simulink model "networkanalyzer"  (R2012b)
settings: Solver=ode3  SolverMode=SingleTasking  StartTime=0.0  StopTime=50000  RelTol=1e-3
libraries: xbsIndex_r4 x1097, casper_library_flow_control x33, casper_library_misc x21, xps_library x10
(part 2 of 8)

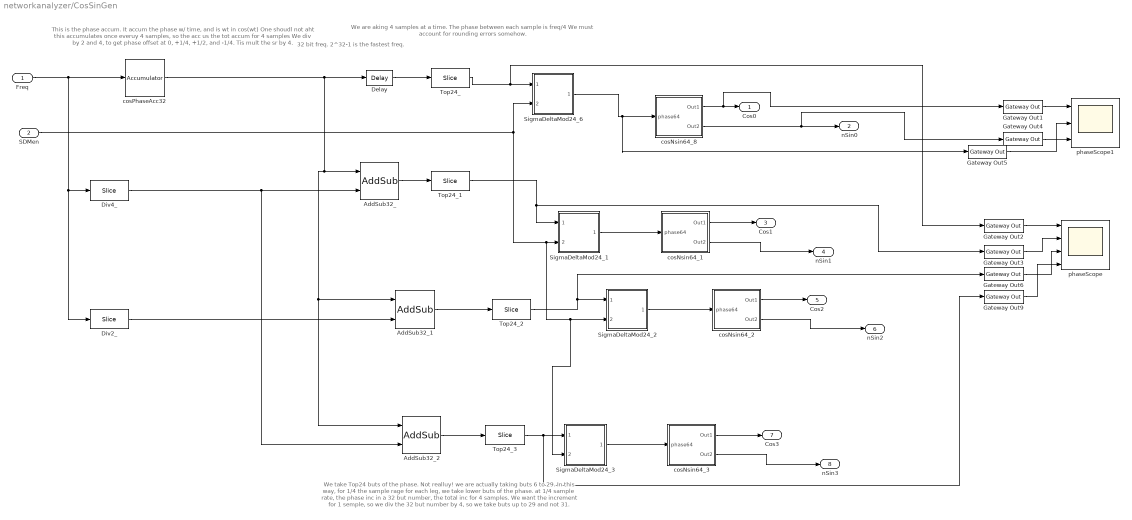
== system networkanalyzer/CosSinGen ==
  note: We take Top24 buts of the phase.
      | Not realluy! we are actually taking buts 6 to 29. In this way,
      | for 1/4 the sample rage for each leg, we take lower buts
      | of the phase. at 1/4 sample rate, the phase inc in a 32 but number,
      | the total inc for 4 samples. We want the increment for 1 semple, so
      | we div the 32 but number by 4, so we take buts up to 29 and not 31.
  note: This is the phase accum. It accum the phase w/ time, and is wt in cos(wt)
      | One shoudl not aht this accumulates once everuy 4 samples, so the acc us the tot accum for 4 samples
      | We div by 2 and 4, to get phase offset at 0, +1/4, +1/2, and -1/4. Tis mult the sr by 4.
  note: 32 bit freq. 2^32-1 is the fastest freq.
  note: We are aking 4 samples at a time.
      | The phase between each sample is freq/4
      | We must account for rounding errors somehow.
  Freq : Inport
  SDMen : Inport  Port=2
  AddSub32_ : xbsIndex_r4/AddSub  mode=Addition  use_carryin=off  use_carryout=off  en=off  latency=2  precision=User Defined  arith_type=Unsigned  n_bits=32  bin_pt=0  quantization=Truncate  overflow=Wrap  dbl_ovrd=off  use_behavioral_HDL=off  hw_selection=Fabric  pipelined=off  block_type=addsub
  AddSub32_1 : xbsIndex_r4/AddSub  mode=Addition  use_carryin=off  use_carryout=off  en=off  latency=2  precision=User Defined  arith_type=Unsigned  n_bits=32  bin_pt=0  quantization=Truncate  overflow=Wrap  dbl_ovrd=off  use_behavioral_HDL=off  hw_selection=Fabric  pipelined=off  block_type=addsub
  AddSub32_2 : xbsIndex_r4/AddSub  mode=Subtraction  use_carryin=off  use_carryout=off  en=off  latency=2  precision=User Defined  arith_type=Unsigned  n_bits=32  bin_pt=0  quantization=Truncate  overflow=Wrap  dbl_ovrd=off  use_behavioral_HDL=off  hw_selection=Fabric  pipelined=off  block_type=addsub
  Delay : xbsIndex_r4/Delay  rst=off  infoeditControl=Selection of Reset will increase slice count due to use of real FFs and instead of SRLs  en=off  latency=2  dbl_ovrd=off  reg_retiming=off  block_type=delay
  Div2_ : xbsIndex_r4/Slice  nbits=31  boolean_output=off  mode=Two Bit Locations  bit1=0  base1=MSB of Input  bit0=1  base0=LSB of Input  dbl_ovrd=off  block_type=slice
  Div4_ : xbsIndex_r4/Slice  nbits=30  boolean_output=off  mode=Two Bit Locations  bit1=0  base1=MSB of Input  bit0=2  base0=LSB of Input  dbl_ovrd=off  block_type=slice
  Gateway Out{1..6,9} (7 alike) : xbsIndex_r4/Gateway Out  inherit_from_input=off  hdl_port=off  timing_constraint=None  locs_specified=off  LOCs={}  UseAsDAC=off  DACChannel='1'  block_type=gatewayout
  SigmaDeltaMod24_1 : Subsystem
  SigmaDeltaMod24_2 : Subsystem
  SigmaDeltaMod24_3 : Subsystem
  SigmaDeltaMod24_6 : Subsystem
  Top24_{,1..3} (4 alike) : xbsIndex_r4/Slice  nbits=24  boolean_output=off  mode=Two Bit Locations  bit1=0  base1=MSB of Input  bit0=6  base0=LSB of Input  dbl_ovrd=off  block_type=slice
  cosNsin64_1 : Subsystem
  cosNsin64_2 : Subsystem
  cosNsin64_3 : Subsystem
  cosNsin64_8 : Subsystem
  cosPhaseAcc32 : xbsIndex_r4/Accumulator  operation=Add  n_bits=32  overflow=Wrap  scale=1  rst=off  hasbypass=off  en=off  dbl_ovrd=off  use_behavioral_HDL=on  implementation=Fabric  block_type=accum
  phaseScope : Scope  NumInputPorts=4
      settings: TimeRange=5000  YMin=0~-5~-5~-5  YMax=300000~5~5~5  SaveName=ScopeData3  MaxDataPoints=10000
  phaseScope1 : Scope  NumInputPorts=3
      settings: TimeRange=5000  YMin=0~-5~-5  YMax=300000~5~5  SaveName=ScopeData6  MaxDataPoints=10000
  Cos0 : Outport
  nSin0 : Outport  Port=2
  Cos1 : Outport  Port=3
  nSin1 : Outport  Port=4
  Cos2 : Outport  Port=5
  nSin2 : Outport  Port=6
  Cos3 : Outport  Port=7
  nSin3 : Outport  Port=8
  wires:
  cosNsin64_1/1(Out1) -> Cos1/1
  cosNsin64_8/2(Out2) -> Gateway Out4/1, nSin0/1
  SigmaDeltaMod24_6/1(DataOut) -> Gateway Out5/1, cosNsin64_8/1(phase64)
  cosNsin64_1/2(Out2) -> nSin1/1
  SDMen/1 -> SigmaDeltaMod24_1/2(SDMEn), SigmaDeltaMod24_3/2(SDMEn), SigmaDeltaMod24_2/2(SDMEn), SigmaDeltaMod24_6/2(SDMEn)
  SigmaDeltaMod24_1/1(DataOut) -> cosNsin64_1/1(phase64)
  Freq/1 -> cosPhaseAcc32/1, Div2_/1, Div4_/1
  Top24_/1 -> Gateway Out2/1, SigmaDeltaMod24_6/1(DataIn)
  cosNsin64_2/1(Out1) -> Cos2/1
  cosNsin64_2/2(Out2) -> nSin2/1
  Top24_2/1 -> SigmaDeltaMod24_2/1(DataIn), Gateway Out6/1
  cosNsin64_3/1(Out1) -> Cos3/1
  cosNsin64_3/2(Out2) -> nSin3/1
  SigmaDeltaMod24_3/1(DataOut) -> cosNsin64_3/1(phase64)
  cosPhaseAcc32/1 -> Delay/1, AddSub32_1/1, AddSub32_2/1, AddSub32_/1
  Div4_/1 -> AddSub32_2/2, AddSub32_/2
  AddSub32_/1 -> Top24_1/1
  Top24_1/1 -> SigmaDeltaMod24_1/1(DataIn), Gateway Out3/1
  AddSub32_1/1 -> Top24_2/1
  Div2_/1 -> AddSub32_1/2
  Delay/1 -> Top24_/1
  AddSub32_2/1 -> Top24_3/1
  Gateway Out2/1 -> phaseScope/1
  Gateway Out3/1 -> phaseScope/2
  Gateway Out6/1 -> phaseScope/3
  Gateway Out9/1 -> phaseScope/4
  SigmaDeltaMod24_2/1(DataOut) -> cosNsin64_2/1(phase64)
  Top24_3/1 -> SigmaDeltaMod24_3/1(DataIn), Gateway Out9/1
  cosNsin64_8/1(Out1) -> Gateway Out1/1, Cos0/1
  Gateway Out1/1 -> phaseScope1/1
  Gateway Out4/1 -> phaseScope1/3
  Gateway Out5/1 -> phaseScope1/2

== system networkanalyzer/DFTMem1 ==
  Start : Inport
  Sel : Inport  Port=2
  Src0 : Inport  Port=3
  Src1 : Inport  Port=4
  Src2 : Inport  Port=5
  Src3 : Inport  Port=6
  WE : Inport  Port=7
  WE1 : Inport  Port=8
  Src4 : Inport  Port=9
  Src5 : Inport  Port=10
  Src6 : Inport  Port=11
  Src7 : Inport  Port=12
  Logical : xbsIndex_r4/Logical  logical_function=OR  inputs=2  en=off  latency=0  precision=Full  arith_type=Unsigned  n_bits=16  bin_pt=0  align_bp=on  dbl_ovrd=off  block_type=logical
  MemRecord : Subsystem
  Mux : xbsIndex_r4/Mux  inputs=8  en=off  latency=0  precision=Full  arith_type=Unsigned  n_bits=16  bin_pt=14  quantization=Truncate  overflow=Wrap  dbl_ovrd=off  block_type=mux
  edge_detect : casper_library_misc/edge_detect  edge=Rising  polarity=Active High  x_in=[0 0.08 0.08 0.16 0.16 0.24 0.24 0.32 0.32 0.4]  y_in="[-1 -1  1  1  1  1  1  1  1  1]"  x_out=[0.6 0.68 0.68 0.76 0.76 0.84 0.84 0.92 0.92 1]  y_out="[-1 -1  1  1 -1 -1 -1 -1 -1 -1]"
  Out1 : Outport
  wires:
  Src2/1 -> Mux/4
  Sel/1 -> Mux/1
  edge_detect/1 -> Logical/2
  WE/1 -> Logical/1
  Src0/1 -> Mux/2
  Src1/1 -> Mux/3
  Src3/1 -> Mux/5
  WE1/1 -> edge_detect/1
  MemRecord/1(memDone) -> Out1/1
  Mux/1 -> MemRecord/2(DataIn)
  Start/1 -> MemRecord/1(Start)
  Logical/1 -> MemRecord/3(WE)
  Src4/1 -> Mux/6
  Src5/1 -> Mux/7
  Src6/1 -> Mux/8
  Src7/1 -> Mux/9

== system networkanalyzer/DFTMem2 ==
  Start : Inport
  Sel : Inport  Port=2
  Src0 : Inport  Port=3
  Src1 : Inport  Port=4
  Src2 : Inport  Port=5
  Src3 : Inport  Port=6
  WE : Inport  Port=7
  WE1 : Inport  Port=8
  Src4 : Inport  Port=9
  Src5 : Inport  Port=10
  Src6 : Inport  Port=11
  Src7 : Inport  Port=12
  Logical : xbsIndex_r4/Logical  logical_function=OR  inputs=2  en=off  latency=0  precision=Full  arith_type=Unsigned  n_bits=16  bin_pt=0  align_bp=on  dbl_ovrd=off  block_type=logical
  MemRecord : Subsystem
  Mux : xbsIndex_r4/Mux  inputs=8  en=off  latency=0  precision=Full  arith_type=Unsigned  n_bits=16  bin_pt=14  quantization=Truncate  overflow=Wrap  dbl_ovrd=off  block_type=mux
  edge_detect : casper_library_misc/edge_detect  edge=Rising  polarity=Active High  x_in=[0 0.08 0.08 0.16 0.16 0.24 0.24 0.32 0.32 0.4]  y_in="[-1 -1  1  1  1  1  1  1  1  1]"  x_out=[0.6 0.68 0.68 0.76 0.76 0.84 0.84 0.92 0.92 1]  y_out="[-1 -1  1  1 -1 -1 -1 -1 -1 -1]"
  Out1 : Outport
  wires:
  Src2/1 -> Mux/4
  Sel/1 -> Mux/1
  edge_detect/1 -> Logical/2
  WE/1 -> Logical/1
  Src0/1 -> Mux/2
  Src1/1 -> Mux/3
  Src3/1 -> Mux/5
  WE1/1 -> edge_detect/1
  MemRecord/1(memDone) -> Out1/1
  Mux/1 -> MemRecord/2(DataIn)
  Start/1 -> MemRecord/1(Start)
  Logical/1 -> MemRecord/3(WE)
  Src4/1 -> Mux/6
  Src5/1 -> Mux/7
  Src6/1 -> Mux/8
  Src7/1 -> Mux/9

== system networkanalyzer/DFTMem3 ==
  Start : Inport
  Sel : Inport  Port=2
  Src0 : Inport  Port=3
  Src1 : Inport  Port=4
  Src2 : Inport  Port=5
  Src3 : Inport  Port=6
  WE : Inport  Port=7
  WE1 : Inport  Port=8
  Src4 : Inport  Port=9
  Src5 : Inport  Port=10
  Src6 : Inport  Port=11
  Src7 : Inport  Port=12
  Logical : xbsIndex_r4/Logical  logical_function=OR  inputs=2  en=off  latency=0  precision=Full  arith_type=Unsigned  n_bits=16  bin_pt=0  align_bp=on  dbl_ovrd=off  block_type=logical
  MemRecord : Subsystem
  Mux : xbsIndex_r4/Mux  inputs=8  en=off  latency=0  precision=Full  arith_type=Unsigned  n_bits=16  bin_pt=14  quantization=Truncate  overflow=Wrap  dbl_ovrd=off  block_type=mux
  edge_detect : casper_library_misc/edge_detect  edge=Rising  polarity=Active High  x_in=[0 0.08 0.08 0.16 0.16 0.24 0.24 0.32 0.32 0.4]  y_in="[-1 -1  1  1  1  1  1  1  1  1]"  x_out=[0.6 0.68 0.68 0.76 0.76 0.84 0.84 0.92 0.92 1]  y_out="[-1 -1  1  1 -1 -1 -1 -1 -1 -1]"
  Out1 : Outport
  wires:
  Src2/1 -> Mux/4
  Sel/1 -> Mux/1
  edge_detect/1 -> Logical/2
  WE/1 -> Logical/1
  Src0/1 -> Mux/2
  Src1/1 -> Mux/3
  Src3/1 -> Mux/5
  WE1/1 -> edge_detect/1
  MemRecord/1(memDone) -> Out1/1
  Mux/1 -> MemRecord/2(DataIn)
  Start/1 -> MemRecord/1(Start)
  Logical/1 -> MemRecord/3(WE)
  Src4/1 -> Mux/6
  Src5/1 -> Mux/7
  Src6/1 -> Mux/8
  Src7/1 -> Mux/9

== system networkanalyzer/DFTMem4 ==
  Start : Inport
  Sel : Inport  Port=2
  Src0 : Inport  Port=3
  Src1 : Inport  Port=4
  Src2 : Inport  Port=5
  Src3 : Inport  Port=6
  WE : Inport  Port=7
  WE1 : Inport  Port=8
  Src4 : Inport  Port=9
  Src5 : Inport  Port=10
  Src6 : Inport  Port=11
  Src7 : Inport  Port=12
  Logical : xbsIndex_r4/Logical  logical_function=OR  inputs=2  en=off  latency=0  precision=Full  arith_type=Unsigned  n_bits=16  bin_pt=0  align_bp=on  dbl_ovrd=off  block_type=logical
  MemRecord : Subsystem
  Mux : xbsIndex_r4/Mux  inputs=8  en=off  latency=0  precision=Full  arith_type=Unsigned  n_bits=16  bin_pt=14  quantization=Truncate  overflow=Wrap  dbl_ovrd=off  block_type=mux
  edge_detect : casper_library_misc/edge_detect  edge=Rising  polarity=Active High  x_in=[0 0.08 0.08 0.16 0.16 0.24 0.24 0.32 0.32 0.4]  y_in="[-1 -1  1  1  1  1  1  1  1  1]"  x_out=[0.6 0.68 0.68 0.76 0.76 0.84 0.84 0.92 0.92 1]  y_out="[-1 -1  1  1 -1 -1 -1 -1 -1 -1]"
  Out1 : Outport
  wires:
  Src2/1 -> Mux/4
  Sel/1 -> Mux/1
  edge_detect/1 -> Logical/2
  WE/1 -> Logical/1
  Src0/1 -> Mux/2
  Src1/1 -> Mux/3
  Src3/1 -> Mux/5
  WE1/1 -> edge_detect/1
  MemRecord/1(memDone) -> Out1/1
  Mux/1 -> MemRecord/2(DataIn)
  Start/1 -> MemRecord/1(Start)
  Logical/1 -> MemRecord/3(WE)
  Src4/1 -> Mux/6
  Src5/1 -> Mux/7
  Src6/1 -> Mux/8
  Src7/1 -> Mux/9

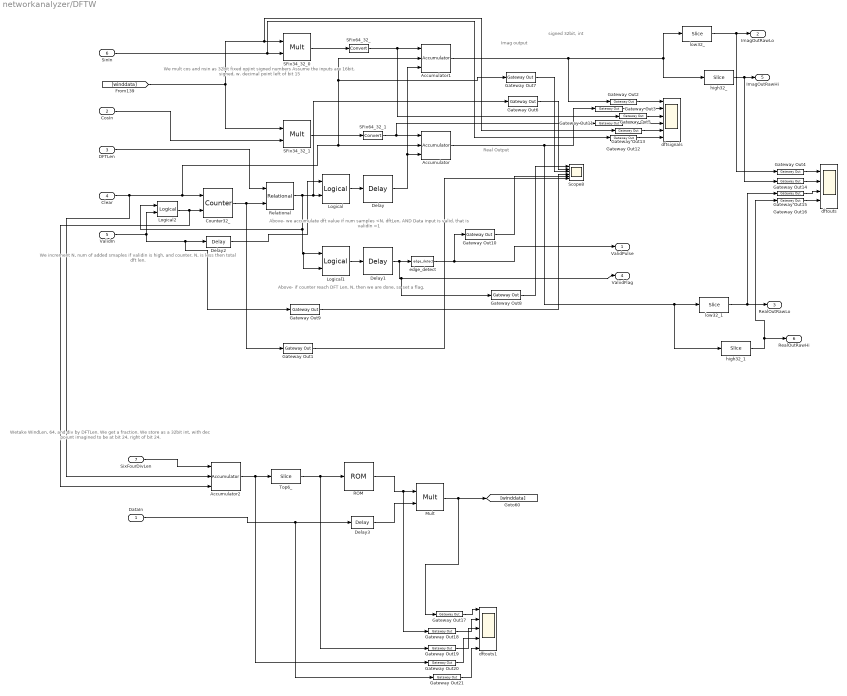
== system networkanalyzer/DFTW ==
  note: Wetake WindLen, 64, and div by DFTLen.
      | We get a fraction. We store as a 32bit int, with dec poiunt imagined to
      | be at bit 24, right of bit 24.
  note: Real Output
  note: Imag output
  note: We mult cos and nsin as 32bit fixed opjint signed numbers
      | Assume the inputs are 16bit, signed, w. decimal point left of bit 15
  note: Above- if counter reach DFT Len, N, then we are done, so set a flag.
  note: Above- we accumulate dft value if num samples <N, dftLen, AND
      | Data input is valid, that is validIn =1
  note: We increment N, num of added smaples if validin is high, and
      | counter, N, is less then total dft len.
  note: signed 32bit, int
  DataIn : Inport
  CosIn : Inport  Port=2
  DFTLen : Inport  Port=3
  Clear : Inport  Port=4
  ValidIn : Inport  Port=5
  SinIn : Inport  Port=6
  SixFourDivLen : Inport  Port=7
  Accumulator : xbsIndex_r4/Accumulator  operation=Add  n_bits=64  overflow=Wrap  scale=1  rst=on  hasbypass=off  en=on  dbl_ovrd=off  use_behavioral_HDL=on  implementation=Fabric  block_type=accum
  Accumulator1 : xbsIndex_r4/Accumulator  operation=Add  n_bits=64  overflow=Wrap  scale=1  rst=on  hasbypass=off  en=on  dbl_ovrd=off  use_behavioral_HDL=on  implementation=Fabric  block_type=accum
  Accumulator2 : xbsIndex_r4/Accumulator  operation=Add  n_bits=32  overflow=Wrap  scale=1  rst=on  hasbypass=off  en=on  dbl_ovrd=off  use_behavioral_HDL=on  implementation=Fabric  block_type=accum
  Counter32_ : xbsIndex_r4/Counter  cnt_type=Free Running  cnt_to=Inf  operation=Up  start_count=0  cnt_by_val=1  arith_type=Unsigned  n_bits=32  bin_pt=0  load_pin=off  rst=on  en=on  explicit_period=on  period=1  dbl_ovrd=off  use_behavioral_HDL=off  implementation=Fabric  block_type=counter
  Delay : xbsIndex_r4/Delay  rst=off  infoeditControl=Selection of Reset will increase slice count due to use of real FFs and instead of SRLs  en=off  latency=2  dbl_ovrd=off  reg_retiming=off  block_type=delay
  Delay1 : xbsIndex_r4/Delay  rst=off  infoeditControl=Selection of Reset will increase slice count due to use of real FFs and instead of SRLs  en=off  latency=2  dbl_ovrd=off  reg_retiming=off  block_type=delay
  Delay2 : xbsIndex_r4/Delay  rst=off  infoeditControl=Selection of Reset will increase slice count due to use of real FFs and instead of SRLs  en=off  latency=2  dbl_ovrd=off  reg_retiming=off  block_type=delay
  Delay3 : xbsIndex_r4/Delay  rst=off  infoeditControl=Selection of Reset will increase slice count due to use of real FFs and instead of SRLs  en=off  latency=1  dbl_ovrd=off  reg_retiming=off  block_type=delay
  Gateway Out{1..21} (21 alike) : xbsIndex_r4/Gateway Out  inherit_from_input=off  hdl_port=off  timing_constraint=None  locs_specified=off  LOCs={}  UseAsDAC=off  DACChannel='1'  block_type=gatewayout
  Logical : xbsIndex_r4/Logical  logical_function=AND  inputs=2  en=off  latency=1  precision=Full  arith_type=Unsigned  n_bits=16  bin_pt=0  align_bp=on  dbl_ovrd=off  block_type=logical
  Logical1 : xbsIndex_r4/Logical  logical_function=NAND  inputs=2  en=off  latency=1  precision=Full  arith_type=Unsigned  n_bits=16  bin_pt=0  align_bp=on  dbl_ovrd=off  block_type=logical
  Logical2 : xbsIndex_r4/Logical  logical_function=AND  inputs=2  en=off  latency=0  precision=Full  arith_type=Unsigned  n_bits=16  bin_pt=0  align_bp=on  dbl_ovrd=off  block_type=logical
  Mult : xbsIndex_r4/Mult  precision=User Defined  arith_type="Signed  (2's comp)"  n_bits=16  bin_pt=15  quantization=Truncate  overflow=Wrap  en=off  latency=3  dbl_ovrd=off  use_behavioral_HDL=off  opt=Speed  use_embedded=on  optimum_pipeline=off  pipeline=on  use_rpm=on  placement_style=Triangular  block_type=mult
  ROM : xbsIndex_r4/ROM  depth=64  initVector=0.5-0.5*cos(2*pi*(0:63)/63)  distributed_mem=Block RAM  rst=off  init_reg=0  en=off  latency=1  gui_display_data_type=Fixed-point  arith_type="Signed  (2's comp)"  n_bits=16  bin_pt=15  preci_type=Single  exp_width=8  frac_width=24  dbl_ovrd=off  optimize=Area  use_rpm=on  block_type=sprom
  Relational : xbsIndex_r4/Relational  mode=a>=b  en=off  latency=1  dbl_ovrd=off  block_type=relational
  SFix34_32_0 : xbsIndex_r4/Mult  precision=User Defined  arith_type="Signed  (2's comp)"  n_bits=34  bin_pt=32  quantization=Truncate  overflow=Saturate  en=off  latency=4  dbl_ovrd=off  use_behavioral_HDL=off  opt=Speed  use_embedded=on  optimum_pipeline=off  pipeline=on  use_rpm=on  placement_style=Triangular  block_type=mult
  SFix34_32_1 : xbsIndex_r4/Mult  precision=User Defined  arith_type="Signed  (2's comp)"  n_bits=34  bin_pt=32  quantization=Truncate  overflow=Saturate  en=off  latency=4  dbl_ovrd=off  use_behavioral_HDL=off  opt=Speed  use_embedded=on  optimum_pipeline=off  pipeline=on  use_rpm=on  placement_style=Triangular  block_type=mult
  SFix64_32_ : xbsIndex_r4/Convert  gui_display_data_type=Fixed-point  arith_type="Signed  (2's comp)"  n_bits=64  bin_pt=32  float_type=Single  exp_bits=8  fraction_bits=24  quantization=Truncate  overflow=Wrap  en=off  latency=0  dbl_ovrd=off  pipeline=off  block_type=convert
  SFix64_32_1 : xbsIndex_r4/Convert  gui_display_data_type=Fixed-point  arith_type="Signed  (2's comp)"  n_bits=64  bin_pt=32  float_type=Single  exp_bits=8  fraction_bits=24  quantization=Truncate  overflow=Wrap  en=off  latency=0  dbl_ovrd=off  pipeline=off  block_type=convert
  Scope8 : Scope  NumInputPorts=6
      settings: YMin=0~-5~-5~-5~-5~-5  YMax=300000~5~5~5~5~5  SaveName=ScopeData18  MaxDataPoints=10000
  Top6_ : xbsIndex_r4/Slice  nbits=6  boolean_output=off  mode=Upper Bit Location + Width  bit1=0  base1=MSB of Input  bit0=0  base0=LSB of Input  dbl_ovrd=off  block_type=slice
  dftouts : Scope  NumInputPorts=4
      settings: YMin=0~-5~-5~-5  YMax=300000~5~5~5  SaveName=ScopeData5  MaxDataPoints=10000
  dftouts1 : Scope  NumInputPorts=5
      settings: YMin=-1~0~0~0~-1  YMax=5.55112e-17~1~70~5e+09~0  MaxDataPoints=10000
  dftsignals : Scope  NumInputPorts=6
      settings: YMin=0~-5~-5~-5~-5~-5  YMax=300000~5~5~5~5~5  SaveName=ScopeData4  MaxDataPoints=10000
  edge_detect : casper_library_misc/edge_detect  edge=Rising  polarity=Active High  x_in=[0 0.08 0.08 0.16 0.16 0.24 0.24 0.32 0.32 0.4]  y_in="[-1 -1  1  1  1  1  1  1  1  1]"  x_out=[0.6 0.68 0.68 0.76 0.76 0.84 0.84 0.92 0.92 1]  y_out="[-1 -1  1  1 -1 -1 -1 -1 -1 -1]"
  high32_ : xbsIndex_r4/Slice  nbits=32  boolean_output=off  mode=Lower Bit Location + Width  bit1=-32  base1=MSB of Input  bit0=32  base0=LSB of Input  dbl_ovrd=off  block_type=slice
  high32_1 : xbsIndex_r4/Slice  nbits=32  boolean_output=off  mode=Lower Bit Location + Width  bit1=-31  base1=MSB of Input  bit0=32  base0=LSB of Input  dbl_ovrd=off  block_type=slice
  low32_ : xbsIndex_r4/Slice  nbits=32  boolean_output=off  mode=Lower Bit Location + Width  bit1=-31  base1=MSB of Input  bit0=0  base0=LSB of Input  dbl_ovrd=off  block_type=slice
  low32_1 : xbsIndex_r4/Slice  nbits=32  boolean_output=off  mode=Lower Bit Location + Width  bit1=-31  base1=MSB of Input  bit0=0  base0=LSB of Input  dbl_ovrd=off  block_type=slice
  ValidPulse : Outport
  ImagOutRawLo : Outport  Port=2
  RealOutRawLo : Outport  Port=3
  ValiidFlag : Outport  Port=4
  ImagOutRawHi : Outport  Port=5
  RealOutRawHi : Outport  Port=6
  wires:
  SFix34_32_1/1 -> SFix64_32_1/1
  Relational/1 -> Logical2/1, Logical1/2, Logical1/1, Gateway Out6/1, Logical/2
  Counter32_/1 -> Gateway Out1/1, Relational/2
  [winddata] -> SFix34_32_1/1, Gateway Out13/1, SFix34_32_0/1
  CosIn/1 -> SFix34_32_1/2
  DFTLen/1 -> Relational/1
  ValidIn/1 -> Logical2/2, Gateway Out9/1, Delay2/1
  Clear/1 -> Accumulator2/2, Gateway Out7/1, Accumulator1/2, Accumulator/2, Counter32_/1
  SinIn/1 -> Gateway Out12/1, SFix34_32_0/2
  Logical/1 -> Delay/1
  Delay/1 -> Accumulator1/3, Accumulator/3
  Logical1/1 -> Delay1/1
  Delay1/1 -> Gateway Out8/1, ValiidFlag/1, edge_detect/1
  edge_detect/1 -> Gateway Out10/1, ValidPulse/1
  Gateway Out6/1 -> Scope8/2
  Gateway Out7/1 -> Scope8/3
  Gateway Out8/1 -> Scope8/1
  Gateway Out9/1 -> Scope8/4
  Gateway Out10/1 -> Scope8/5
  Gateway Out1/1 -> Scope8/6
  Logical2/1 -> Accumulator2/3, Counter32_/2
  Delay2/1 -> Logical/1
  SFix34_32_0/1 -> SFix64_32_/1
  Gateway Out2/1 -> dftsignals/1
  Gateway Out3/1 -> dftsignals/2
  Gateway Out5/1 -> dftsignals/3
  Gateway Out13/1 -> dftsignals/5
  Gateway Out11/1 -> dftsignals/4
  Gateway Out12/1 -> dftsignals/6
  SFix64_32_/1 -> Gateway Out5/1, Accumulator1/1
  SFix64_32_1/1 -> Gateway Out11/1, Accumulator/1
  Accumulator1/1 -> Gateway Out2/1, high32_/1, low32_/1
  Accumulator/1 -> high32_1/1, low32_1/1, Gateway Out3/1
  low32_/1 -> Gateway Out4/1, ImagOutRawLo/1
  high32_/1 -> Gateway Out14/1, ImagOutRawHi/1
  low32_1/1 -> Gateway Out15/1, RealOutRawLo/1
  high32_1/1 -> Gateway Out16/1, RealOutRawHi/1
  Gateway Out15/1 -> dftouts/3
  Gateway Out16/1 -> dftouts/4
  Gateway Out14/1 -> dftouts/2
  Gateway Out4/1 -> dftouts/1
  ROM/1 -> Gateway Out18/1, Mult/1
  Delay3/1 -> Mult/2
  Mult/1 -> Gateway Out17/1, [winddata]
  Top6_/1 -> Gateway Out19/1, ROM/1
  Accumulator2/1 -> Gateway Out20/1, Top6_/1
  SixFourDivLen/1 -> Accumulator2/1
  DataIn/1 -> Gateway Out21/1, Delay3/1
  Gateway Out17/1 -> dftouts1/1
  Gateway Out18/1 -> dftouts1/2
  Gateway Out19/1 -> dftouts1/3
  Gateway Out20/1 -> dftouts1/4
  Gateway Out21/1 -> dftouts1/5

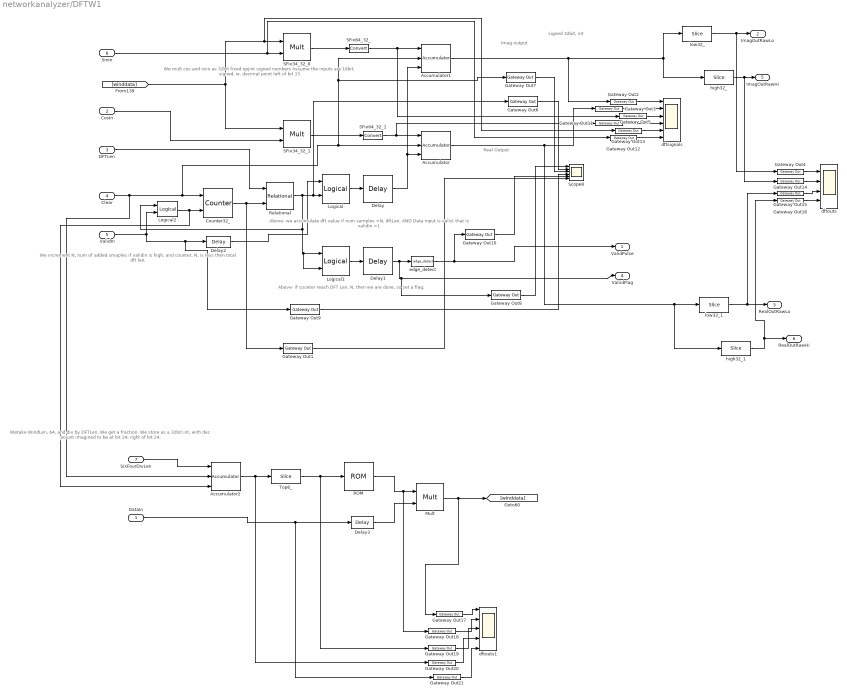
== system networkanalyzer/DFTW1 ==
  note: Wetake WindLen, 64, and div by DFTLen.
      | We get a fraction. We store as a 32bit int, with dec poiunt imagined to
      | be at bit 24, right of bit 24.
  note: Real Output
  note: Imag output
  note: We mult cos and nsin as 32bit fixed opjint signed numbers
      | Assume the inputs are 16bit, signed, w. decimal point left of bit 15
  note: Above- if counter reach DFT Len, N, then we are done, so set a flag.
  note: Above- we accumulate dft value if num samples <N, dftLen, AND
      | Data input is valid, that is validIn =1
  note: We increment N, num of added smaples if validin is high, and
      | counter, N, is less then total dft len.
  note: signed 32bit, int
  DataIn : Inport
  CosIn : Inport  Port=2
  DFTLen : Inport  Port=3
  Clear : Inport  Port=4
  ValidIn : Inport  Port=5
  SinIn : Inport  Port=6
  SixFourDivLen : Inport  Port=7
  Accumulator : xbsIndex_r4/Accumulator  operation=Add  n_bits=64  overflow=Wrap  scale=1  rst=on  hasbypass=off  en=on  dbl_ovrd=off  use_behavioral_HDL=on  implementation=Fabric  block_type=accum
  Accumulator1 : xbsIndex_r4/Accumulator  operation=Add  n_bits=64  overflow=Wrap  scale=1  rst=on  hasbypass=off  en=on  dbl_ovrd=off  use_behavioral_HDL=on  implementation=Fabric  block_type=accum
  Accumulator2 : xbsIndex_r4/Accumulator  operation=Add  n_bits=32  overflow=Wrap  scale=1  rst=on  hasbypass=off  en=on  dbl_ovrd=off  use_behavioral_HDL=on  implementation=Fabric  block_type=accum
  Counter32_ : xbsIndex_r4/Counter  cnt_type=Free Running  cnt_to=Inf  operation=Up  start_count=0  cnt_by_val=1  arith_type=Unsigned  n_bits=32  bin_pt=0  load_pin=off  rst=on  en=on  explicit_period=on  period=1  dbl_ovrd=off  use_behavioral_HDL=off  implementation=Fabric  block_type=counter
  Delay : xbsIndex_r4/Delay  rst=off  infoeditControl=Selection of Reset will increase slice count due to use of real FFs and instead of SRLs  en=off  latency=2  dbl_ovrd=off  reg_retiming=off  block_type=delay
  Delay1 : xbsIndex_r4/Delay  rst=off  infoeditControl=Selection of Reset will increase slice count due to use of real FFs and instead of SRLs  en=off  latency=2  dbl_ovrd=off  reg_retiming=off  block_type=delay
  Delay2 : xbsIndex_r4/Delay  rst=off  infoeditControl=Selection of Reset will increase slice count due to use of real FFs and instead of SRLs  en=off  latency=2  dbl_ovrd=off  reg_retiming=off  block_type=delay
  Delay3 : xbsIndex_r4/Delay  rst=off  infoeditControl=Selection of Reset will increase slice count due to use of real FFs and instead of SRLs  en=off  latency=1  dbl_ovrd=off  reg_retiming=off  block_type=delay
  Gateway Out{1..21} (21 alike) : xbsIndex_r4/Gateway Out  inherit_from_input=off  hdl_port=off  timing_constraint=None  locs_specified=off  LOCs={}  UseAsDAC=off  DACChannel='1'  block_type=gatewayout
  Logical : xbsIndex_r4/Logical  logical_function=AND  inputs=2  en=off  latency=1  precision=Full  arith_type=Unsigned  n_bits=16  bin_pt=0  align_bp=on  dbl_ovrd=off  block_type=logical
  Logical1 : xbsIndex_r4/Logical  logical_function=NAND  inputs=2  en=off  latency=1  precision=Full  arith_type=Unsigned  n_bits=16  bin_pt=0  align_bp=on  dbl_ovrd=off  block_type=logical
  Logical2 : xbsIndex_r4/Logical  logical_function=AND  inputs=2  en=off  latency=0  precision=Full  arith_type=Unsigned  n_bits=16  bin_pt=0  align_bp=on  dbl_ovrd=off  block_type=logical
  Mult : xbsIndex_r4/Mult  precision=User Defined  arith_type="Signed  (2's comp)"  n_bits=16  bin_pt=15  quantization=Truncate  overflow=Wrap  en=off  latency=3  dbl_ovrd=off  use_behavioral_HDL=off  opt=Speed  use_embedded=on  optimum_pipeline=off  pipeline=on  use_rpm=on  placement_style=Triangular  block_type=mult
  ROM : xbsIndex_r4/ROM  depth=64  initVector=0.5-0.5*cos(2*pi*(0:63)/63)  distributed_mem=Block RAM  rst=off  init_reg=0  en=off  latency=1  gui_display_data_type=Fixed-point  arith_type="Signed  (2's comp)"  n_bits=16  bin_pt=15  preci_type=Single  exp_width=8  frac_width=24  dbl_ovrd=off  optimize=Area  use_rpm=on  block_type=sprom
  Relational : xbsIndex_r4/Relational  mode=a>=b  en=off  latency=1  dbl_ovrd=off  block_type=relational
  SFix34_32_0 : xbsIndex_r4/Mult  precision=User Defined  arith_type="Signed  (2's comp)"  n_bits=34  bin_pt=32  quantization=Truncate  overflow=Saturate  en=off  latency=4  dbl_ovrd=off  use_behavioral_HDL=off  opt=Speed  use_embedded=on  optimum_pipeline=off  pipeline=on  use_rpm=on  placement_style=Triangular  block_type=mult
  SFix34_32_1 : xbsIndex_r4/Mult  precision=User Defined  arith_type="Signed  (2's comp)"  n_bits=34  bin_pt=32  quantization=Truncate  overflow=Saturate  en=off  latency=4  dbl_ovrd=off  use_behavioral_HDL=off  opt=Speed  use_embedded=on  optimum_pipeline=off  pipeline=on  use_rpm=on  placement_style=Triangular  block_type=mult
  SFix64_32_ : xbsIndex_r4/Convert  gui_display_data_type=Fixed-point  arith_type="Signed  (2's comp)"  n_bits=64  bin_pt=32  float_type=Single  exp_bits=8  fraction_bits=24  quantization=Truncate  overflow=Wrap  en=off  latency=0  dbl_ovrd=off  pipeline=off  block_type=convert
  SFix64_32_1 : xbsIndex_r4/Convert  gui_display_data_type=Fixed-point  arith_type="Signed  (2's comp)"  n_bits=64  bin_pt=32  float_type=Single  exp_bits=8  fraction_bits=24  quantization=Truncate  overflow=Wrap  en=off  latency=0  dbl_ovrd=off  pipeline=off  block_type=convert
  Scope8 : Scope  NumInputPorts=6
      settings: YMin=0~-5~-5~-5~-5~-5  YMax=300000~5~5~5~5~5  SaveName=ScopeData18  MaxDataPoints=10000
  Top6_ : xbsIndex_r4/Slice  nbits=6  boolean_output=off  mode=Upper Bit Location + Width  bit1=0  base1=MSB of Input  bit0=0  base0=LSB of Input  dbl_ovrd=off  block_type=slice
  dftouts : Scope  NumInputPorts=4
      settings: YMin=0~-5~-5~-5  YMax=300000~5~5~5  SaveName=ScopeData5  MaxDataPoints=10000
  dftouts1 : Scope  NumInputPorts=5
      settings: YMin=-1~0~0~0~-1  YMax=5.55112e-17~1~70~5e+09~0  MaxDataPoints=10000
  dftsignals : Scope  NumInputPorts=6
      settings: YMin=0~-5~-5~-5~-5~-5  YMax=300000~5~5~5~5~5  SaveName=ScopeData4  MaxDataPoints=10000
  edge_detect : casper_library_misc/edge_detect  edge=Rising  polarity=Active High  x_in=[0 0.08 0.08 0.16 0.16 0.24 0.24 0.32 0.32 0.4]  y_in="[-1 -1  1  1  1  1  1  1  1  1]"  x_out=[0.6 0.68 0.68 0.76 0.76 0.84 0.84 0.92 0.92 1]  y_out="[-1 -1  1  1 -1 -1 -1 -1 -1 -1]"
  high32_ : xbsIndex_r4/Slice  nbits=32  boolean_output=off  mode=Lower Bit Location + Width  bit1=-32  base1=MSB of Input  bit0=32  base0=LSB of Input  dbl_ovrd=off  block_type=slice
  high32_1 : xbsIndex_r4/Slice  nbits=32  boolean_output=off  mode=Lower Bit Location + Width  bit1=-31  base1=MSB of Input  bit0=32  base0=LSB of Input  dbl_ovrd=off  block_type=slice
  low32_ : xbsIndex_r4/Slice  nbits=32  boolean_output=off  mode=Lower Bit Location + Width  bit1=-31  base1=MSB of Input  bit0=0  base0=LSB of Input  dbl_ovrd=off  block_type=slice
  low32_1 : xbsIndex_r4/Slice  nbits=32  boolean_output=off  mode=Lower Bit Location + Width  bit1=-31  base1=MSB of Input  bit0=0  base0=LSB of Input  dbl_ovrd=off  block_type=slice
  ValidPulse : Outport
  ImagOutRawLo : Outport  Port=2
  RealOutRawLo : Outport  Port=3
  ValiidFlag : Outport  Port=4
  ImagOutRawHi : Outport  Port=5
  RealOutRawHi : Outport  Port=6
  wires:
  SFix34_32_1/1 -> SFix64_32_1/1
  Relational/1 -> Logical2/1, Logical1/2, Logical1/1, Gateway Out6/1, Logical/2
  Counter32_/1 -> Gateway Out1/1, Relational/2
  [winddata] -> SFix34_32_1/1, Gateway Out13/1, SFix34_32_0/1
  CosIn/1 -> SFix34_32_1/2
  DFTLen/1 -> Relational/1
  ValidIn/1 -> Logical2/2, Gateway Out9/1, Delay2/1
  Clear/1 -> Accumulator2/2, Gateway Out7/1, Accumulator1/2, Accumulator/2, Counter32_/1
  SinIn/1 -> Gateway Out12/1, SFix34_32_0/2
  Logical/1 -> Delay/1
  Delay/1 -> Accumulator1/3, Accumulator/3
  Logical1/1 -> Delay1/1
  Delay1/1 -> Gateway Out8/1, ValiidFlag/1, edge_detect/1
  edge_detect/1 -> Gateway Out10/1, ValidPulse/1
  Gateway Out6/1 -> Scope8/2
  Gateway Out7/1 -> Scope8/3
  Gateway Out8/1 -> Scope8/1
  Gateway Out9/1 -> Scope8/4
  Gateway Out10/1 -> Scope8/5
  Gateway Out1/1 -> Scope8/6
  Logical2/1 -> Accumulator2/3, Counter32_/2
  Delay2/1 -> Logical/1
  SFix34_32_0/1 -> SFix64_32_/1
  Gateway Out2/1 -> dftsignals/1
  Gateway Out3/1 -> dftsignals/2
  Gateway Out5/1 -> dftsignals/3
  Gateway Out13/1 -> dftsignals/5
  Gateway Out11/1 -> dftsignals/4
  Gateway Out12/1 -> dftsignals/6
  SFix64_32_/1 -> Gateway Out5/1, Accumulator1/1
  SFix64_32_1/1 -> Gateway Out11/1, Accumulator/1
  Accumulator1/1 -> Gateway Out2/1, high32_/1, low32_/1
  Accumulator/1 -> high32_1/1, low32_1/1, Gateway Out3/1
  low32_/1 -> Gateway Out4/1, ImagOutRawLo/1
  high32_/1 -> Gateway Out14/1, ImagOutRawHi/1
  low32_1/1 -> Gateway Out15/1, RealOutRawLo/1
  high32_1/1 -> Gateway Out16/1, RealOutRawHi/1
  Gateway Out15/1 -> dftouts/3
  Gateway Out16/1 -> dftouts/4
  Gateway Out14/1 -> dftouts/2
  Gateway Out4/1 -> dftouts/1
  ROM/1 -> Gateway Out18/1, Mult/1
  Delay3/1 -> Mult/2
  Mult/1 -> Gateway Out17/1, [winddata]
  Top6_/1 -> Gateway Out19/1, ROM/1
  Accumulator2/1 -> Gateway Out20/1, Top6_/1
  SixFourDivLen/1 -> Accumulator2/1
  DataIn/1 -> Gateway Out21/1, Delay3/1
  Gateway Out17/1 -> dftouts1/1
  Gateway Out18/1 -> dftouts1/2
  Gateway Out19/1 -> dftouts1/3
  Gateway Out20/1 -> dftouts1/4
  Gateway Out21/1 -> dftouts1/5

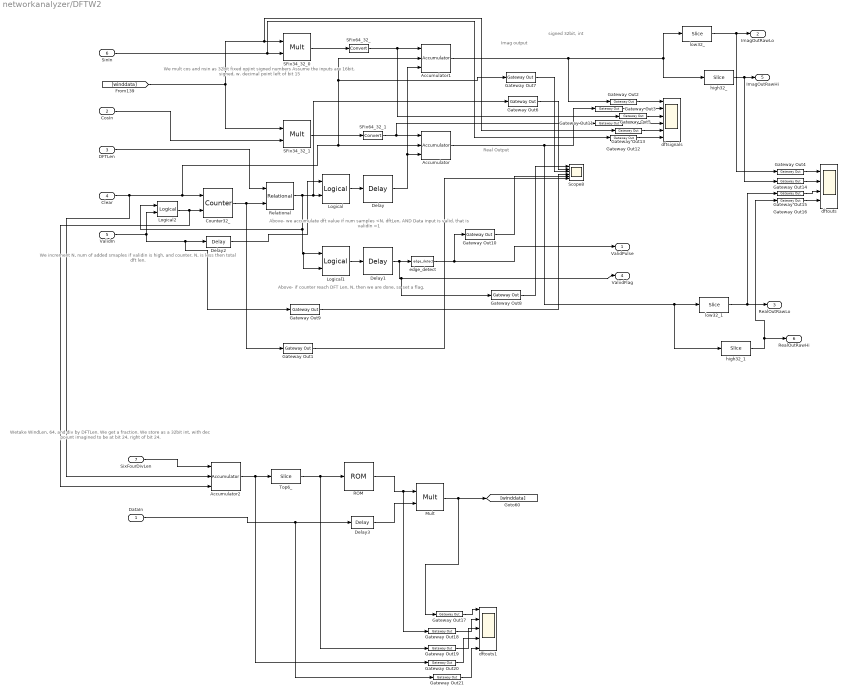
== system networkanalyzer/DFTW2 ==
  note: Wetake WindLen, 64, and div by DFTLen.
      | We get a fraction. We store as a 32bit int, with dec poiunt imagined to
      | be at bit 24, right of bit 24.
  note: Real Output
  note: Imag output
  note: We mult cos and nsin as 32bit fixed opjint signed numbers
      | Assume the inputs are 16bit, signed, w. decimal point left of bit 15
  note: Above- if counter reach DFT Len, N, then we are done, so set a flag.
  note: Above- we accumulate dft value if num samples <N, dftLen, AND
      | Data input is valid, that is validIn =1
  note: We increment N, num of added smaples if validin is high, and
      | counter, N, is less then total dft len.
  note: signed 32bit, int
  DataIn : Inport
  CosIn : Inport  Port=2
  DFTLen : Inport  Port=3
  Clear : Inport  Port=4
  ValidIn : Inport  Port=5
  SinIn : Inport  Port=6
  SixFourDivLen : Inport  Port=7
  Accumulator : xbsIndex_r4/Accumulator  operation=Add  n_bits=64  overflow=Wrap  scale=1  rst=on  hasbypass=off  en=on  dbl_ovrd=off  use_behavioral_HDL=on  implementation=Fabric  block_type=accum
  Accumulator1 : xbsIndex_r4/Accumulator  operation=Add  n_bits=64  overflow=Wrap  scale=1  rst=on  hasbypass=off  en=on  dbl_ovrd=off  use_behavioral_HDL=on  implementation=Fabric  block_type=accum
  Accumulator2 : xbsIndex_r4/Accumulator  operation=Add  n_bits=32  overflow=Wrap  scale=1  rst=on  hasbypass=off  en=on  dbl_ovrd=off  use_behavioral_HDL=on  implementation=Fabric  block_type=accum
  Counter32_ : xbsIndex_r4/Counter  cnt_type=Free Running  cnt_to=Inf  operation=Up  start_count=0  cnt_by_val=1  arith_type=Unsigned  n_bits=32  bin_pt=0  load_pin=off  rst=on  en=on  explicit_period=on  period=1  dbl_ovrd=off  use_behavioral_HDL=off  implementation=Fabric  block_type=counter
  Delay : xbsIndex_r4/Delay  rst=off  infoeditControl=Selection of Reset will increase slice count due to use of real FFs and instead of SRLs  en=off  latency=2  dbl_ovrd=off  reg_retiming=off  block_type=delay
  Delay1 : xbsIndex_r4/Delay  rst=off  infoeditControl=Selection of Reset will increase slice count due to use of real FFs and instead of SRLs  en=off  latency=2  dbl_ovrd=off  reg_retiming=off  block_type=delay
  Delay2 : xbsIndex_r4/Delay  rst=off  infoeditControl=Selection of Reset will increase slice count due to use of real FFs and instead of SRLs  en=off  latency=2  dbl_ovrd=off  reg_retiming=off  block_type=delay
  Delay3 : xbsIndex_r4/Delay  rst=off  infoeditControl=Selection of Reset will increase slice count due to use of real FFs and instead of SRLs  en=off  latency=1  dbl_ovrd=off  reg_retiming=off  block_type=delay
  Gateway Out{1..21} (21 alike) : xbsIndex_r4/Gateway Out  inherit_from_input=off  hdl_port=off  timing_constraint=None  locs_specified=off  LOCs={}  UseAsDAC=off  DACChannel='1'  block_type=gatewayout
  Logical : xbsIndex_r4/Logical  logical_function=AND  inputs=2  en=off  latency=1  precision=Full  arith_type=Unsigned  n_bits=16  bin_pt=0  align_bp=on  dbl_ovrd=off  block_type=logical
  Logical1 : xbsIndex_r4/Logical  logical_function=NAND  inputs=2  en=off  latency=1  precision=Full  arith_type=Unsigned  n_bits=16  bin_pt=0  align_bp=on  dbl_ovrd=off  block_type=logical
  Logical2 : xbsIndex_r4/Logical  logical_function=AND  inputs=2  en=off  latency=0  precision=Full  arith_type=Unsigned  n_bits=16  bin_pt=0  align_bp=on  dbl_ovrd=off  block_type=logical
  Mult : xbsIndex_r4/Mult  precision=User Defined  arith_type="Signed  (2's comp)"  n_bits=16  bin_pt=15  quantization=Truncate  overflow=Wrap  en=off  latency=3  dbl_ovrd=off  use_behavioral_HDL=off  opt=Speed  use_embedded=on  optimum_pipeline=off  pipeline=on  use_rpm=on  placement_style=Triangular  block_type=mult
  ROM : xbsIndex_r4/ROM  depth=64  initVector=0.5-0.5*cos(2*pi*(0:63)/63)  distributed_mem=Block RAM  rst=off  init_reg=0  en=off  latency=1  gui_display_data_type=Fixed-point  arith_type="Signed  (2's comp)"  n_bits=16  bin_pt=15  preci_type=Single  exp_width=8  frac_width=24  dbl_ovrd=off  optimize=Area  use_rpm=on  block_type=sprom
  Relational : xbsIndex_r4/Relational  mode=a>=b  en=off  latency=1  dbl_ovrd=off  block_type=relational
  SFix34_32_0 : xbsIndex_r4/Mult  precision=User Defined  arith_type="Signed  (2's comp)"  n_bits=34  bin_pt=32  quantization=Truncate  overflow=Saturate  en=off  latency=4  dbl_ovrd=off  use_behavioral_HDL=off  opt=Speed  use_embedded=on  optimum_pipeline=off  pipeline=on  use_rpm=on  placement_style=Triangular  block_type=mult
  SFix34_32_1 : xbsIndex_r4/Mult  precision=User Defined  arith_type="Signed  (2's comp)"  n_bits=34  bin_pt=32  quantization=Truncate  overflow=Saturate  en=off  latency=4  dbl_ovrd=off  use_behavioral_HDL=off  opt=Speed  use_embedded=on  optimum_pipeline=off  pipeline=on  use_rpm=on  placement_style=Triangular  block_type=mult
  SFix64_32_ : xbsIndex_r4/Convert  gui_display_data_type=Fixed-point  arith_type="Signed  (2's comp)"  n_bits=64  bin_pt=32  float_type=Single  exp_bits=8  fraction_bits=24  quantization=Truncate  overflow=Wrap  en=off  latency=0  dbl_ovrd=off  pipeline=off  block_type=convert
  SFix64_32_1 : xbsIndex_r4/Convert  gui_display_data_type=Fixed-point  arith_type="Signed  (2's comp)"  n_bits=64  bin_pt=32  float_type=Single  exp_bits=8  fraction_bits=24  quantization=Truncate  overflow=Wrap  en=off  latency=0  dbl_ovrd=off  pipeline=off  block_type=convert
  Scope8 : Scope  NumInputPorts=6
      settings: YMin=0~-5~-5~-5~-5~-5  YMax=300000~5~5~5~5~5  SaveName=ScopeData18  MaxDataPoints=10000
  Top6_ : xbsIndex_r4/Slice  nbits=6  boolean_output=off  mode=Upper Bit Location + Width  bit1=0  base1=MSB of Input  bit0=0  base0=LSB of Input  dbl_ovrd=off  block_type=slice
  dftouts : Scope  NumInputPorts=4
      settings: YMin=0~-5~-5~-5  YMax=300000~5~5~5  SaveName=ScopeData5  MaxDataPoints=10000
  dftouts1 : Scope  NumInputPorts=5
      settings: YMin=-1~0~0~0~-1  YMax=5.55112e-17~1~70~5e+09~0  MaxDataPoints=10000
  dftsignals : Scope  NumInputPorts=6
      settings: YMin=0~-5~-5~-5~-5~-5  YMax=300000~5~5~5~5~5  SaveName=ScopeData4  MaxDataPoints=10000
  edge_detect : casper_library_misc/edge_detect  edge=Rising  polarity=Active High  x_in=[0 0.08 0.08 0.16 0.16 0.24 0.24 0.32 0.32 0.4]  y_in="[-1 -1  1  1  1  1  1  1  1  1]"  x_out=[0.6 0.68 0.68 0.76 0.76 0.84 0.84 0.92 0.92 1]  y_out="[-1 -1  1  1 -1 -1 -1 -1 -1 -1]"
  high32_ : xbsIndex_r4/Slice  nbits=32  boolean_output=off  mode=Lower Bit Location + Width  bit1=-32  base1=MSB of Input  bit0=32  base0=LSB of Input  dbl_ovrd=off  block_type=slice
  high32_1 : xbsIndex_r4/Slice  nbits=32  boolean_output=off  mode=Lower Bit Location + Width  bit1=-31  base1=MSB of Input  bit0=32  base0=LSB of Input  dbl_ovrd=off  block_type=slice
  low32_ : xbsIndex_r4/Slice  nbits=32  boolean_output=off  mode=Lower Bit Location + Width  bit1=-31  base1=MSB of Input  bit0=0  base0=LSB of Input  dbl_ovrd=off  block_type=slice
  low32_1 : xbsIndex_r4/Slice  nbits=32  boolean_output=off  mode=Lower Bit Location + Width  bit1=-31  base1=MSB of Input  bit0=0  base0=LSB of Input  dbl_ovrd=off  block_type=slice
  ValidPulse : Outport
  ImagOutRawLo : Outport  Port=2
  RealOutRawLo : Outport  Port=3
  ValiidFlag : Outport  Port=4
  ImagOutRawHi : Outport  Port=5
  RealOutRawHi : Outport  Port=6
  wires:
  SFix34_32_1/1 -> SFix64_32_1/1
  Relational/1 -> Logical2/1, Logical1/2, Logical1/1, Gateway Out6/1, Logical/2
  Counter32_/1 -> Gateway Out1/1, Relational/2
  [winddata] -> SFix34_32_1/1, Gateway Out13/1, SFix34_32_0/1
  CosIn/1 -> SFix34_32_1/2
  DFTLen/1 -> Relational/1
  ValidIn/1 -> Logical2/2, Gateway Out9/1, Delay2/1
  Clear/1 -> Accumulator2/2, Gateway Out7/1, Accumulator1/2, Accumulator/2, Counter32_/1
  SinIn/1 -> Gateway Out12/1, SFix34_32_0/2
  Logical/1 -> Delay/1
  Delay/1 -> Accumulator1/3, Accumulator/3
  Logical1/1 -> Delay1/1
  Delay1/1 -> Gateway Out8/1, ValiidFlag/1, edge_detect/1
  edge_detect/1 -> Gateway Out10/1, ValidPulse/1
  Gateway Out6/1 -> Scope8/2
  Gateway Out7/1 -> Scope8/3
  Gateway Out8/1 -> Scope8/1
  Gateway Out9/1 -> Scope8/4
  Gateway Out10/1 -> Scope8/5
  Gateway Out1/1 -> Scope8/6
  Logical2/1 -> Accumulator2/3, Counter32_/2
  Delay2/1 -> Logical/1
  SFix34_32_0/1 -> SFix64_32_/1
  Gateway Out2/1 -> dftsignals/1
  Gateway Out3/1 -> dftsignals/2
  Gateway Out5/1 -> dftsignals/3
  Gateway Out13/1 -> dftsignals/5
  Gateway Out11/1 -> dftsignals/4
  Gateway Out12/1 -> dftsignals/6
  SFix64_32_/1 -> Gateway Out5/1, Accumulator1/1
  SFix64_32_1/1 -> Gateway Out11/1, Accumulator/1
  Accumulator1/1 -> Gateway Out2/1, high32_/1, low32_/1
  Accumulator/1 -> high32_1/1, low32_1/1, Gateway Out3/1
  low32_/1 -> Gateway Out4/1, ImagOutRawLo/1
  high32_/1 -> Gateway Out14/1, ImagOutRawHi/1
  low32_1/1 -> Gateway Out15/1, RealOutRawLo/1
  high32_1/1 -> Gateway Out16/1, RealOutRawHi/1
  Gateway Out15/1 -> dftouts/3
  Gateway Out16/1 -> dftouts/4
  Gateway Out14/1 -> dftouts/2
  Gateway Out4/1 -> dftouts/1
  ROM/1 -> Gateway Out18/1, Mult/1
  Delay3/1 -> Mult/2
  Mult/1 -> Gateway Out17/1, [winddata]
  Top6_/1 -> Gateway Out19/1, ROM/1
  Accumulator2/1 -> Gateway Out20/1, Top6_/1
  SixFourDivLen/1 -> Accumulator2/1
  DataIn/1 -> Gateway Out21/1, Delay3/1
  Gateway Out17/1 -> dftouts1/1
  Gateway Out18/1 -> dftouts1/2
  Gateway Out19/1 -> dftouts1/3
  Gateway Out20/1 -> dftouts1/4
  Gateway Out21/1 -> dftouts1/5

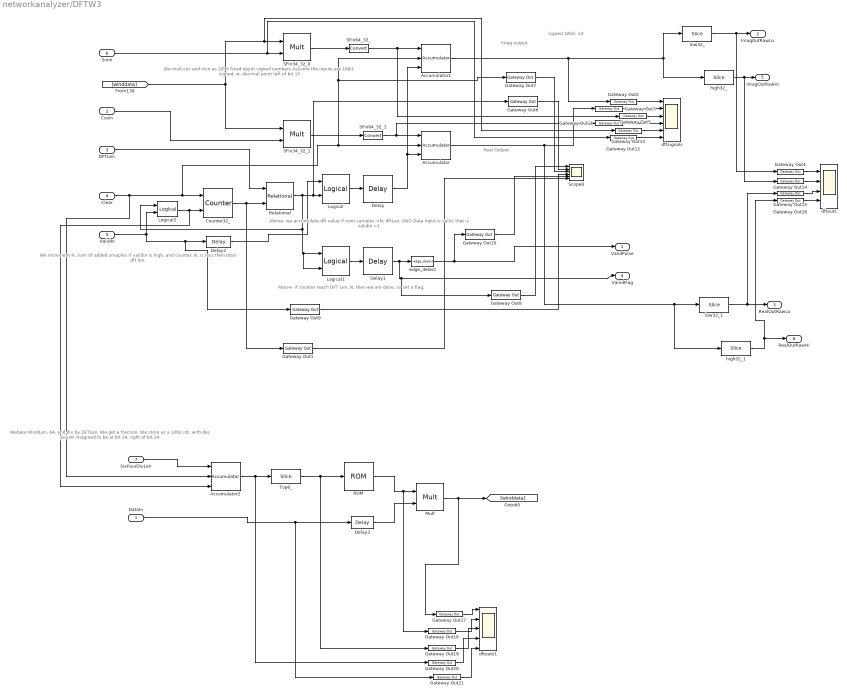
== system networkanalyzer/DFTW3 ==
  note: Wetake WindLen, 64, and div by DFTLen.
      | We get a fraction. We store as a 32bit int, with dec poiunt imagined to
      | be at bit 24, right of bit 24.
  note: Real Output
  note: Imag output
  note: We mult cos and nsin as 32bit fixed opjint signed numbers
      | Assume the inputs are 16bit, signed, w. decimal point left of bit 15
  note: Above- if counter reach DFT Len, N, then we are done, so set a flag.
  note: Above- we accumulate dft value if num samples <N, dftLen, AND
      | Data input is valid, that is validIn =1
  note: We increment N, num of added smaples if validin is high, and
      | counter, N, is less then total dft len.
  note: signed 32bit, int
  DataIn : Inport
  CosIn : Inport  Port=2
  DFTLen : Inport  Port=3
  Clear : Inport  Port=4
  ValidIn : Inport  Port=5
  SinIn : Inport  Port=6
  SixFourDivLen : Inport  Port=7
  Accumulator : xbsIndex_r4/Accumulator  operation=Add  n_bits=64  overflow=Wrap  scale=1  rst=on  hasbypass=off  en=on  dbl_ovrd=off  use_behavioral_HDL=on  implementation=Fabric  block_type=accum
  Accumulator1 : xbsIndex_r4/Accumulator  operation=Add  n_bits=64  overflow=Wrap  scale=1  rst=on  hasbypass=off  en=on  dbl_ovrd=off  use_behavioral_HDL=on  implementation=Fabric  block_type=accum
  Accumulator2 : xbsIndex_r4/Accumulator  operation=Add  n_bits=32  overflow=Wrap  scale=1  rst=on  hasbypass=off  en=on  dbl_ovrd=off  use_behavioral_HDL=on  implementation=Fabric  block_type=accum
  Counter32_ : xbsIndex_r4/Counter  cnt_type=Free Running  cnt_to=Inf  operation=Up  start_count=0  cnt_by_val=1  arith_type=Unsigned  n_bits=32  bin_pt=0  load_pin=off  rst=on  en=on  explicit_period=on  period=1  dbl_ovrd=off  use_behavioral_HDL=off  implementation=Fabric  block_type=counter
  Delay : xbsIndex_r4/Delay  rst=off  infoeditControl=Selection of Reset will increase slice count due to use of real FFs and instead of SRLs  en=off  latency=2  dbl_ovrd=off  reg_retiming=off  block_type=delay
  Delay1 : xbsIndex_r4/Delay  rst=off  infoeditControl=Selection of Reset will increase slice count due to use of real FFs and instead of SRLs  en=off  latency=2  dbl_ovrd=off  reg_retiming=off  block_type=delay
  Delay2 : xbsIndex_r4/Delay  rst=off  infoeditControl=Selection of Reset will increase slice count due to use of real FFs and instead of SRLs  en=off  latency=2  dbl_ovrd=off  reg_retiming=off  block_type=delay
  Delay3 : xbsIndex_r4/Delay  rst=off  infoeditControl=Selection of Reset will increase slice count due to use of real FFs and instead of SRLs  en=off  latency=1  dbl_ovrd=off  reg_retiming=off  block_type=delay
  Gateway Out{1..21} (21 alike) : xbsIndex_r4/Gateway Out  inherit_from_input=off  hdl_port=off  timing_constraint=None  locs_specified=off  LOCs={}  UseAsDAC=off  DACChannel='1'  block_type=gatewayout
  Logical : xbsIndex_r4/Logical  logical_function=AND  inputs=2  en=off  latency=1  precision=Full  arith_type=Unsigned  n_bits=16  bin_pt=0  align_bp=on  dbl_ovrd=off  block_type=logical
  Logical1 : xbsIndex_r4/Logical  logical_function=NAND  inputs=2  en=off  latency=1  precision=Full  arith_type=Unsigned  n_bits=16  bin_pt=0  align_bp=on  dbl_ovrd=off  block_type=logical
  Logical2 : xbsIndex_r4/Logical  logical_function=AND  inputs=2  en=off  latency=0  precision=Full  arith_type=Unsigned  n_bits=16  bin_pt=0  align_bp=on  dbl_ovrd=off  block_type=logical
  Mult : xbsIndex_r4/Mult  precision=User Defined  arith_type="Signed  (2's comp)"  n_bits=16  bin_pt=15  quantization=Truncate  overflow=Wrap  en=off  latency=3  dbl_ovrd=off  use_behavioral_HDL=off  opt=Speed  use_embedded=on  optimum_pipeline=off  pipeline=on  use_rpm=on  placement_style=Triangular  block_type=mult
  ROM : xbsIndex_r4/ROM  depth=64  initVector=0.5-0.5*cos(2*pi*(0:63)/63)  distributed_mem=Block RAM  rst=off  init_reg=0  en=off  latency=1  gui_display_data_type=Fixed-point  arith_type="Signed  (2's comp)"  n_bits=16  bin_pt=15  preci_type=Single  exp_width=8  frac_width=24  dbl_ovrd=off  optimize=Area  use_rpm=on  block_type=sprom
  Relational : xbsIndex_r4/Relational  mode=a>=b  en=off  latency=1  dbl_ovrd=off  block_type=relational
  SFix34_32_0 : xbsIndex_r4/Mult  precision=User Defined  arith_type="Signed  (2's comp)"  n_bits=34  bin_pt=32  quantization=Truncate  overflow=Saturate  en=off  latency=4  dbl_ovrd=off  use_behavioral_HDL=off  opt=Speed  use_embedded=on  optimum_pipeline=off  pipeline=on  use_rpm=on  placement_style=Triangular  block_type=mult
  SFix34_32_1 : xbsIndex_r4/Mult  precision=User Defined  arith_type="Signed  (2's comp)"  n_bits=34  bin_pt=32  quantization=Truncate  overflow=Saturate  en=off  latency=4  dbl_ovrd=off  use_behavioral_HDL=off  opt=Speed  use_embedded=on  optimum_pipeline=off  pipeline=on  use_rpm=on  placement_style=Triangular  block_type=mult
  SFix64_32_ : xbsIndex_r4/Convert  gui_display_data_type=Fixed-point  arith_type="Signed  (2's comp)"  n_bits=64  bin_pt=32  float_type=Single  exp_bits=8  fraction_bits=24  quantization=Truncate  overflow=Wrap  en=off  latency=0  dbl_ovrd=off  pipeline=off  block_type=convert
  SFix64_32_1 : xbsIndex_r4/Convert  gui_display_data_type=Fixed-point  arith_type="Signed  (2's comp)"  n_bits=64  bin_pt=32  float_type=Single  exp_bits=8  fraction_bits=24  quantization=Truncate  overflow=Wrap  en=off  latency=0  dbl_ovrd=off  pipeline=off  block_type=convert
  Scope8 : Scope  NumInputPorts=6
      settings: YMin=0~-5~-5~-5~-5~-5  YMax=300000~5~5~5~5~5  SaveName=ScopeData18  MaxDataPoints=10000
  Top6_ : xbsIndex_r4/Slice  nbits=6  boolean_output=off  mode=Upper Bit Location + Width  bit1=0  base1=MSB of Input  bit0=0  base0=LSB of Input  dbl_ovrd=off  block_type=slice
  dftouts : Scope  NumInputPorts=4
      settings: YMin=0~-5~-5~-5  YMax=300000~5~5~5  SaveName=ScopeData5  MaxDataPoints=10000
  dftouts1 : Scope  NumInputPorts=5
      settings: YMin=-1~0~0~0~-1  YMax=5.55112e-17~1~70~5e+09~0  MaxDataPoints=10000
  dftsignals : Scope  NumInputPorts=6
      settings: YMin=0~-5~-5~-5~-5~-5  YMax=300000~5~5~5~5~5  SaveName=ScopeData4  MaxDataPoints=10000
  edge_detect : casper_library_misc/edge_detect  edge=Rising  polarity=Active High  x_in=[0 0.08 0.08 0.16 0.16 0.24 0.24 0.32 0.32 0.4]  y_in="[-1 -1  1  1  1  1  1  1  1  1]"  x_out=[0.6 0.68 0.68 0.76 0.76 0.84 0.84 0.92 0.92 1]  y_out="[-1 -1  1  1 -1 -1 -1 -1 -1 -1]"
  high32_ : xbsIndex_r4/Slice  nbits=32  boolean_output=off  mode=Lower Bit Location + Width  bit1=-32  base1=MSB of Input  bit0=32  base0=LSB of Input  dbl_ovrd=off  block_type=slice
  high32_1 : xbsIndex_r4/Slice  nbits=32  boolean_output=off  mode=Lower Bit Location + Width  bit1=-31  base1=MSB of Input  bit0=32  base0=LSB of Input  dbl_ovrd=off  block_type=slice
  low32_ : xbsIndex_r4/Slice  nbits=32  boolean_output=off  mode=Lower Bit Location + Width  bit1=-31  base1=MSB of Input  bit0=0  base0=LSB of Input  dbl_ovrd=off  block_type=slice
  low32_1 : xbsIndex_r4/Slice  nbits=32  boolean_output=off  mode=Lower Bit Location + Width  bit1=-31  base1=MSB of Input  bit0=0  base0=LSB of Input  dbl_ovrd=off  block_type=slice
  ValidPulse : Outport
  ImagOutRawLo : Outport  Port=2
  RealOutRawLo : Outport  Port=3
  ValiidFlag : Outport  Port=4
  ImagOutRawHi : Outport  Port=5
  RealOutRawHi : Outport  Port=6
  wires:
  SFix34_32_1/1 -> SFix64_32_1/1
  Relational/1 -> Logical2/1, Logical1/2, Logical1/1, Gateway Out6/1, Logical/2
  Counter32_/1 -> Gateway Out1/1, Relational/2
  [winddata] -> SFix34_32_1/1, Gateway Out13/1, SFix34_32_0/1
  CosIn/1 -> SFix34_32_1/2
  DFTLen/1 -> Relational/1
  ValidIn/1 -> Logical2/2, Gateway Out9/1, Delay2/1
  Clear/1 -> Accumulator2/2, Gateway Out7/1, Accumulator1/2, Accumulator/2, Counter32_/1
  SinIn/1 -> Gateway Out12/1, SFix34_32_0/2
  Logical/1 -> Delay/1
  Delay/1 -> Accumulator1/3, Accumulator/3
  Logical1/1 -> Delay1/1
  Delay1/1 -> Gateway Out8/1, ValiidFlag/1, edge_detect/1
  edge_detect/1 -> Gateway Out10/1, ValidPulse/1
  Gateway Out6/1 -> Scope8/2
  Gateway Out7/1 -> Scope8/3
  Gateway Out8/1 -> Scope8/1
  Gateway Out9/1 -> Scope8/4
  Gateway Out10/1 -> Scope8/5
  Gateway Out1/1 -> Scope8/6
  Logical2/1 -> Accumulator2/3, Counter32_/2
  Delay2/1 -> Logical/1
  SFix34_32_0/1 -> SFix64_32_/1
  Gateway Out2/1 -> dftsignals/1
  Gateway Out3/1 -> dftsignals/2
  Gateway Out5/1 -> dftsignals/3
  Gateway Out13/1 -> dftsignals/5
  Gateway Out11/1 -> dftsignals/4
  Gateway Out12/1 -> dftsignals/6
  SFix64_32_/1 -> Gateway Out5/1, Accumulator1/1
  SFix64_32_1/1 -> Gateway Out11/1, Accumulator/1
  Accumulator1/1 -> Gateway Out2/1, high32_/1, low32_/1
  Accumulator/1 -> high32_1/1, low32_1/1, Gateway Out3/1
  low32_/1 -> Gateway Out4/1, ImagOutRawLo/1
  high32_/1 -> Gateway Out14/1, ImagOutRawHi/1
  low32_1/1 -> Gateway Out15/1, RealOutRawLo/1
  high32_1/1 -> Gateway Out16/1, RealOutRawHi/1
  Gateway Out15/1 -> dftouts/3
  Gateway Out16/1 -> dftouts/4
  Gateway Out14/1 -> dftouts/2
  Gateway Out4/1 -> dftouts/1
  ROM/1 -> Gateway Out18/1, Mult/1
  Delay3/1 -> Mult/2
  Mult/1 -> Gateway Out17/1, [winddata]
  Top6_/1 -> Gateway Out19/1, ROM/1
  Accumulator2/1 -> Gateway Out20/1, Top6_/1
  SixFourDivLen/1 -> Accumulator2/1
  DataIn/1 -> Gateway Out21/1, Delay3/1
  Gateway Out17/1 -> dftouts1/1
  Gateway Out18/1 -> dftouts1/2
  Gateway Out19/1 -> dftouts1/3
  Gateway Out20/1 -> dftouts1/4
  Gateway Out21/1 -> dftouts1/5
